simulink model "model"  (R2023b)
settings: Solver=VariableStepAuto  StartTime=0.0  StopTime=10.0  RelTol=1e-3
values from neighbouring files (symbols this model uses):
  a = 1.3    [script.m]
  A = [(-CF-CR)/(m*Vv),(-CF*a+CR*b-m*Vv^2)/(m*Vv^2) ... (first row only)    [script.m]
  b = 1.5    [script.m]
  B = [CF/(m*Vv) CR/(m*Vv) ... (first row only)    [script.m]
  C = [1,0 ... (first row only)    [script.m]
  CF = 2*60000    (= 120000)    [script.m]
  CR = 2*60000    (= 120000)    [script.m]
  D = [0 0 ... (first row only)    [script.m]
  Jz = 2875    [script.m]
  K = place(A_c,B1_c,[-1 -10 -50 -100])    [script.m]
  Kff = ((m*V^2)/l)*(b/CF-a/CR+(a*K(3)/CR))+l-l*K(3)    [script.m]
  m = 1575    [script.m]
  V = Vv    (= 22.2222222222)    [script.m]
  Vv = 80/3.6    (= 22.2222222222)    [script.m]
libraries: simulink_extras x4
settings Model: Creator=dadog  LastModifiedBy=dadog
settings DataIOCC: ReturnWorkspaceOutputs=off

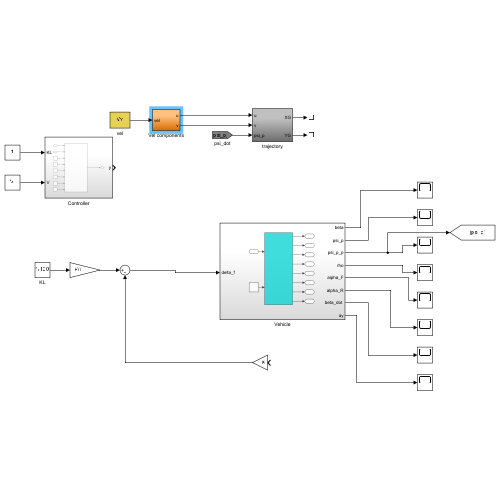
[thumbnail: Simulink's stored preview of the top-level diagram]
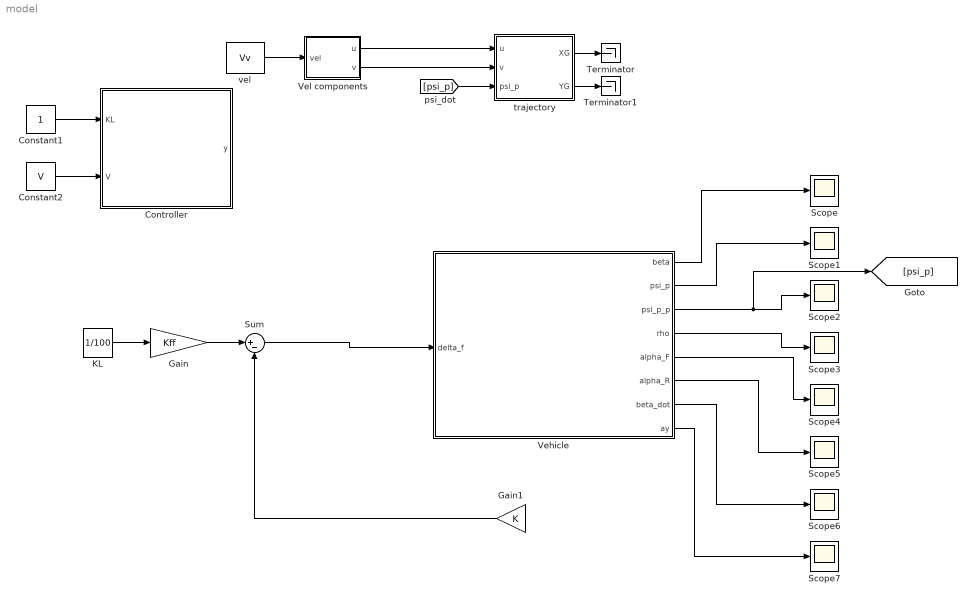
== system model ==
  Constant1 : Constant
  Constant2 : Constant  Value=V
  Controller : Subsystem
  Gain : Gain  Gain=Kff
  Gain1 : Gain  Gain=K
  KL : Constant  Value=1/100
  Scope{,1..7} (8 alike) : Scope
  Sum : Sum  Inputs=|+-
  Terminator : Terminator
  Terminator1 : Terminator
  Vehicle : Subsystem
  Vel components : Subsystem
  trajectory : Subsystem
  vel : Constant  Value=Vv
  wires:
  Sum/1 -> Vehicle/1(delta_f)
  Vehicle/1(beta) -> Scope/1
  Vehicle/2(psi_p) -> Scope1/1
  Vehicle/3(psi_p_p) -> [psi_p], Scope2/1
  Vehicle/4(rho) -> Scope3/1
  Vehicle/5(alpha_F) -> Scope4/1
  Vehicle/6(alpha_R) -> Scope5/1
  Vehicle/7("beta_dot ") -> Scope6/1
  Vehicle/8(ay) -> Scope7/1
  [psi_p] -> trajectory/3(psi_p)
  trajectory/2(YG) -> Terminator1/1
  Vel components/1(u) -> trajectory/1(u)
  trajectory/1(XG) -> Terminator/1
  vel/1 -> Vel components/1(vel)
  Vel components/2(v) -> trajectory/2(v)
  Constant2/1 -> Controller/2(V)
  Constant1/1 -> Controller/1(KL)
  KL/1 -> Gain/1
  Gain/1 -> Sum/1
  Gain1/1 -> Sum/2

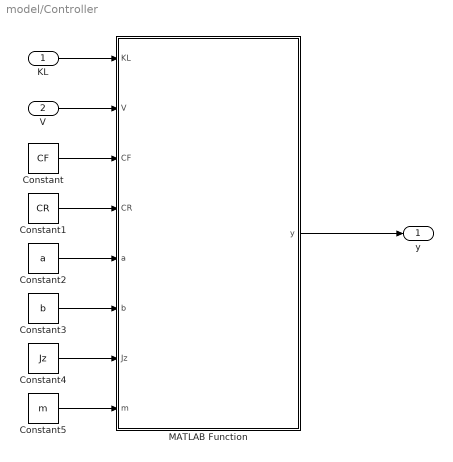
== system model/Controller ==
  KL : Inport
  V : Inport  Port=2
  Constant : Constant  Value=CF
  Constant1 : Constant  Value=CR
  Constant2 : Constant  Value=a
  Constant3 : Constant  Value=b
  Constant4 : Constant  Value=Jz
  Constant5 : Constant  Value=m
  MATLAB Function : MATLAB Function  TreatAsAtomicUnit=on
  y : Outport
  wires:
  KL/1 -> MATLAB Function/1(KL)
  V/1 -> MATLAB Function/2(V)
  MATLAB Function/1(y) -> y/1
  Constant1/1 -> MATLAB Function/4(CR)
  Constant2/1 -> MATLAB Function/5(a)
  Constant/1 -> MATLAB Function/3(CF)
  Constant3/1 -> MATLAB Function/6(b)
  Constant4/1 -> MATLAB Function/7(Jz)
  Constant5/1 -> MATLAB Function/8(m)

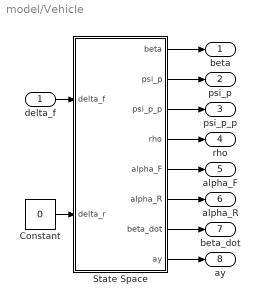
== system model/Vehicle ==
  delta_f : Inport
  Constant : Constant  Value=0
  State Space : Subsystem
  beta : Outport
  psi_p : Outport  Port=2
  psi_p_p : Outport  Port=3
  rho : Outport  Port=4
  alpha_F : Outport  Port=5
  alpha_R : Outport  Port=6
  "beta_dot " : Outport  Port=7
  ay : Outport  Port=8
  wires:
  State Space/6(alpha_R) -> alpha_R/1
  State Space/3(psi_p_p) -> psi_p_p/1
  State Space/1(beta) -> beta/1
  State Space/2(psi_p) -> psi_p/1
  delta_f/1 -> State Space/1(delta_f)
  State Space/7("beta_dot ") -> "beta_dot "/1
  State Space/5(alpha_F) -> alpha_F/1
  State Space/4(rho) -> rho/1
  State Space/8(ay) -> ay/1
  Constant/1 -> State Space/2(delta_r)

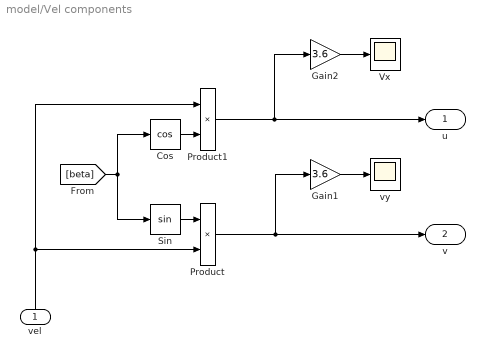
== system model/Vel components ==
  vel : Inport
  Cos : Trigonometry  Operator=cos
  Gain1 : Gain  Gain=3.6
  Gain2 : Gain  Gain=3.6
  Product : Product
  Product1 : Product
  Sin : Trigonometry
  Vx : Scope
  vy : Scope
  u : Outport  VectorParamsAs1DForOutWhenUnconnected=off
  v : Outport  Port=2  VectorParamsAs1DForOutWhenUnconnected=off
  wires:
  Product/1 -> Gain1/1, v/1
  vel/1 -> Product/2, Product1/1
  Gain1/1 -> vy/1
  Gain2/1 -> Vx/1
  Cos/1 -> Product1/2
  Product1/1 -> Gain2/1, u/1
  [beta] -> Sin/1, Cos/1
  Sin/1 -> Product/1

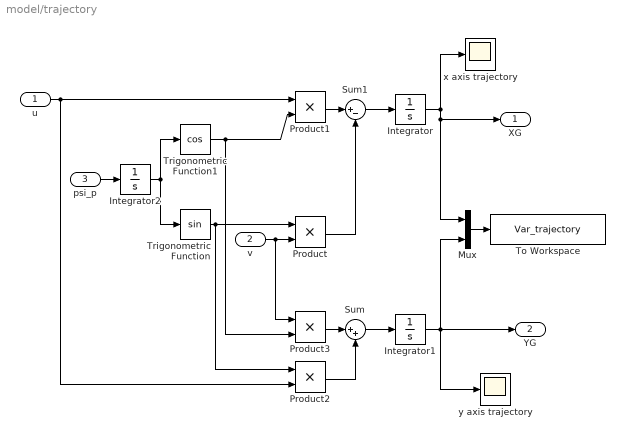
== system model/trajectory ==
  u : Inport
  v : Inport  Port=2
  psi_p : Inport  Port=3
  Integrator : Integrator
  Integrator1 : Integrator
  Integrator2 : Integrator
  Mux : Mux  Inputs=2
  Product{,1..3} (4 alike) : Product  InputSameDT=on  SaturateOnIntegerOverflow=on  OutDataTypeStr=Inherit: Same as first input
  Sum : Sum  Inputs=|++  InputSameDT=on  SaturateOnIntegerOverflow=on  OutDataTypeStr=Inherit: Same as first input
  Sum1 : Sum  Inputs=|+-  InputSameDT=on  SaturateOnIntegerOverflow=on  OutDataTypeStr=Inherit: Same as first input
  To Workspace : ToWorkspace  VariableName=Var_trajectory  SampleTime=-1
      settings: Save2DSignal=2-D array (concatenate along first dimension)
      settings: InitFcn=|
      | ParentName = get_param(gcb,'Parent');
      | cont = max(find(ParentName=='/'));
      | set_param(gcb,'VariableName',strcat('Var_',ParentName(cont+1:length(ParentName))));
      | clear ParentName cont
  Trigonometric Function : Trigonometry
  Trigonometric Function1 : Trigonometry  Operator=cos
  x axis trajectory : Scope
  y axis trajectory : Scope
  XG : Outport  VectorParamsAs1DForOutWhenUnconnected=off
  YG : Outport  Port=2  VectorParamsAs1DForOutWhenUnconnected=off
  wires:
  psi_p/1 -> Integrator2/1
  Product1/1 -> Sum1/1
  Product/1 -> Sum1/2
  Sum1/1 -> Integrator/1
  Trigonometric Function/1 -> Product/1, Product2/1
  u/1 -> Product2/2, Product1/1
  v/1 -> Product/2, Product3/1
  Trigonometric Function1/1 -> Product1/2, Product3/2
  Product3/1 -> Sum/1
  Product2/1 -> Sum/2
  Sum/1 -> Integrator1/1
  Integrator/1 -> XG/1, Mux/1, x axis trajectory/1
  Integrator1/1 -> YG/1, y axis trajectory/1, Mux/2
  Mux/1 -> To Workspace/1
  Integrator2/1 -> Trigonometric Function/1, Trigonometric Function1/1

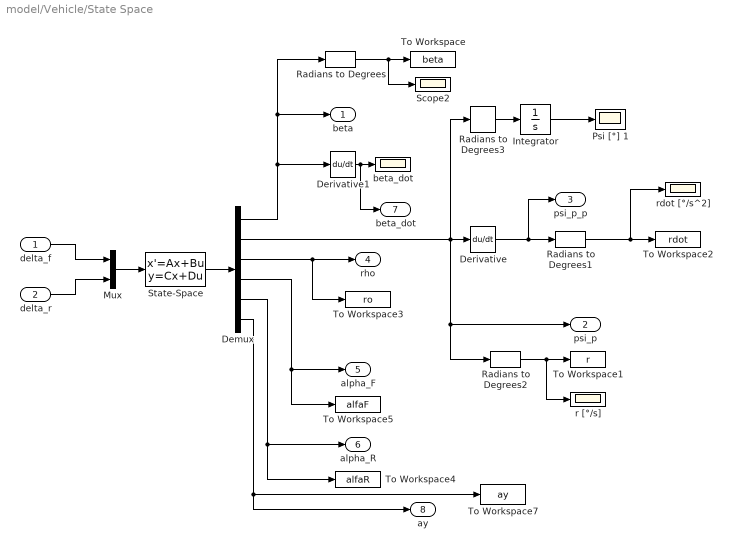
== system model/Vehicle/State Space ==
  delta_f : Inport
  delta_r : Inport  Port=2
  Demux : Demux  Outputs=6
  Derivative : Derivative
  Derivative1 : Derivative
  Integrator : Integrator
  Mux : Mux  Inputs=2
  Psi [°] 1 : Scope
  Radians to Degrees{,1..3} (4 alike) : simulink_extras/Transformations/Radians to Degrees
  Scope2 : Scope
  State-Space : StateSpace  A=A  B=B  C=C  D=D  InitialCondition=0
  To Workspace : ToWorkspace  VariableName=beta  SaveFormat=Timeseries  SampleTime=-1
  To Workspace1 : ToWorkspace  VariableName=r  SaveFormat=Timeseries  SampleTime=-1
  To Workspace2 : ToWorkspace  VariableName=rdot  SaveFormat=Timeseries  SampleTime=-1
  To Workspace3 : ToWorkspace  VariableName=ro  SaveFormat=Timeseries  SampleTime=-1
  To Workspace4 : ToWorkspace  VariableName=alfaR  SaveFormat=Timeseries  SampleTime=-1
  To Workspace5 : ToWorkspace  VariableName=alfaF  SaveFormat=Timeseries  SampleTime=-1
  To Workspace7 : ToWorkspace  VariableName=ay  SaveFormat=Timeseries  SampleTime=-1
      settings: Save2DSignal=2-D array (concatenate along first dimension)
  beta_dot : Scope
  r [°/s] : Scope
  rdot [°/s^2] : Scope
  beta : Outport  VectorParamsAs1DForOutWhenUnconnected=off
  psi_p : Outport  Port=2  VectorParamsAs1DForOutWhenUnconnected=off
  psi_p_p : Outport  Port=3  VectorParamsAs1DForOutWhenUnconnected=off
  rho : Outport  Port=4  VectorParamsAs1DForOutWhenUnconnected=off
  alpha_F : Outport  Port=5  VectorParamsAs1DForOutWhenUnconnected=off
  alpha_R : Outport  Port=6  VectorParamsAs1DForOutWhenUnconnected=off
  "beta_dot " : Outport  Port=7  VectorParamsAs1DForOutWhenUnconnected=off
  ay : Outport  Port=8  VectorParamsAs1DForOutWhenUnconnected=off
  wires:
  Demux/2 -> psi_p/1, Radians to Degrees2/1, Radians to Degrees3/1, Derivative/1
  Demux/1 -> Derivative1/1, beta/1, Radians to Degrees/1
  Derivative/1 -> Radians to Degrees1/1, psi_p_p/1
  Radians to Degrees/1 -> Scope2/1, To Workspace/1
  Radians to Degrees1/1 -> rdot [°/s^2]/1, To Workspace2/1
  Radians to Degrees2/1 -> r [°/s]/1, To Workspace1/1
  Demux/3 -> To Workspace3/1, rho/1
  Demux/4 -> alpha_F/1, To Workspace5/1
  Demux/5 -> To Workspace4/1, alpha_R/1
  Radians to Degrees3/1 -> Integrator/1
  Integrator/1 -> Psi [°] 1/1
  Derivative1/1 -> "beta_dot "/1, beta_dot/1
  delta_f/1 -> Mux/1
  delta_r/1 -> Mux/2
  Demux/6 -> ay/1, To Workspace7/1
  Mux/1 -> State-Space/1
  State-Space/1 -> Demux/1

== matlab function model/Controller/MATLAB Function ==
  data: KL input; y output; V input; CF input; CR input; a input; b input; Jz input; m input
function y = fcn(KL, V, CF, CR, a, b, Jz, m)
% lf = a, lr = b, J_psi = Jz

% State space matrices
% A = [0 1 0 0
%     0 -(CF+CR)/(m*V) (CF+CR)/m (CR*b-CF*a)/(m*V)
%     0 0 0 1
%     0 (CR*b-CF*a)/(Jz*V) (CF*a-CR*b)/Jz -(CR*b^2+CF*a^2)/(Jz*V)];
% 
% B1 = [0
%     CF/m
%     0
%     (CF*a)/Jz];
% 
% B2 = [0
%     ((CR*b-CF*a)/(m*V))-V
%     0
%     -(CR*b^2+CF*a^2)/(Jz*V)];

% C = eye(4);

% Simulink does not see place().
%K=place(A,B1,[-1 -10 -50 -100]);


y = 10;


end
